simulink library "Ampere_Library"  (R2022b)
settings: Solver=FixedStepDiscrete  StartTime=0  StopTime=10.0  RelTol=1e-3  EnableMultiTasking=on
undefined symbols (not defined in the file or in its folder): A_INST_double, Dem_EventStatusType, ECU_AMBIENT_TEMPERATURE, SET_ECU_AMBIENT_TEMPERATURE, SlDemoSign, Std_ReturnType
libraries: simulink x13
(part 8 of 10)

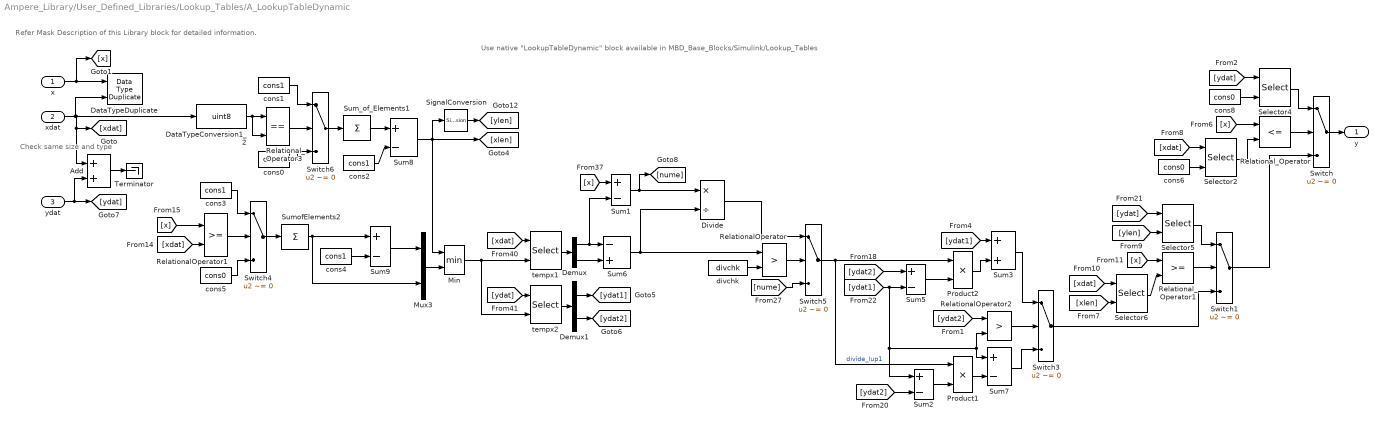
== system Ampere_Library/User_Defined_Libraries/Lookup_Tables/A_LookupTableDynamic ==
  note: Check same size and type
  note: Refer Mask Description of this Library block for detailed information.
  note: Use native "LookupTableDynamic" block available in MBD_Base_Blocks/Simulink/Lookup_Tables
  x : Inport
  xdat : Inport  Port=2
  ydat : Inport  Port=3
  Add : Sum  InputSameDT=on  RndMeth=Zero
  DataTypeConversion1_2 : DataTypeConversion  OutDataTypeStr=uint8
      settings: AttributesFormatString=SAT = %<SaturateOnIntegerOverflow>
  DataTypeDuplicate : DataTypeDuplicate
  Demux : Demux  Outputs=2
  Demux1 : Demux  Outputs=2
  Divide : Product  Inputs=*/  OutDataTypeStr=Inherit: Inherit via back propagation  RndMeth=Zero
      settings: AttributesFormatString=SAT = %<SaturateOnIntegerOverflow>\nDT = %<OutDataTypeStr>\n
  Min : MinMax  Inputs=2  InputSameDT=on  RndMeth=Zero  SaturateOnIntegerOverflow=on
      settings: AttributesFormatString=SAT = %<SaturateOnIntegerOverflow>
  Mux3 : Mux  Inputs=2
  Product1 : Product  OutDataTypeStr=Inherit: Inherit via back propagation  RndMeth=Zero
      settings: AttributesFormatString=SAT = %<SaturateOnIntegerOverflow>\nDT = %<OutDataTypeStr>\n
  Product2 : Product  OutDataTypeStr=Inherit: Inherit via back propagation  RndMeth=Zero
      settings: AttributesFormatString=SAT = %<SaturateOnIntegerOverflow>\nDT = %<OutDataTypeStr>\n
  RelationalOperator : RelationalOperator  Operator=>  OutDataTypeStr=boolean  RndMeth=Zero
  RelationalOperator1 : RelationalOperator  OutDataTypeStr=boolean  RndMeth=Zero
  RelationalOperator2 : RelationalOperator  Operator=>  OutDataTypeStr=boolean  RndMeth=Zero
  Relational_Operator : RelationalOperator  Operator=<=  OutDataTypeStr=boolean  RndMeth=Zero
  Relational_Operator1 : RelationalOperator  OutDataTypeStr=boolean  RndMeth=Zero
  Relational_Operator3 : RelationalOperator  Operator===  OutDataTypeStr=boolean  RndMeth=Zero
  Selector{2,4..6} (4 alike) : Selector  IndexMode=Zero-based  IndexOptions=Index vector (port)  Indices=SelIdx  OutputSizes=1
  SignalConversion : SignalConversion  OverrideOpt=off
  Sum{1..2,5,7} (4 alike) : Sum  Inputs=+-  InputSameDT=on  RndMeth=Zero
      settings: AttributesFormatString=SAT = %<SaturateOnIntegerOverflow>
  Sum3 : Sum  InputSameDT=on  RndMeth=Zero
      settings: AttributesFormatString=SAT = %<SaturateOnIntegerOverflow>
  Sum6 : Sum  Inputs=-+  InputSameDT=on  RndMeth=Zero
      settings: AttributesFormatString=SAT = %<SaturateOnIntegerOverflow>
  Sum8 : Sum  Inputs=+-  InputSameDT=on  RndMeth=Zero  SaturateOnIntegerOverflow=on
      settings: AttributesFormatString=SAT = %<SaturateOnIntegerOverflow>
  Sum9 : Sum  Inputs=+-  InputSameDT=on  RndMeth=Zero  SaturateOnIntegerOverflow=on
      settings: AttributesFormatString=SAT = %<SaturateOnIntegerOverflow>
  Sum_of_Elements1 : Sum  Inputs=+  InputSameDT=on  RndMeth=Zero  SaturateOnIntegerOverflow=on
      settings: AttributesFormatString=SAT = %<SaturateOnIntegerOverflow>
  SumofElements2 : Sum  Inputs=+  InputSameDT=on  RndMeth=Zero  SaturateOnIntegerOverflow=on
      settings: AttributesFormatString=SAT = %<SaturateOnIntegerOverflow>\n
  Switch{,1,3..6} (6 alike) : Switch  Criteria=u2 ~= 0  RndMeth=Zero  SaturateOnIntegerOverflow=off
      settings: AttributesFormatString=SAT = %<SaturateOnIntegerOverflow>
  Terminator : Terminator
  cons{0,5..6,8} (4 alike) : Constant  Value=cons0  OutDataTypeStr=uint8
      cons0 settings: AttributesFormatString=DT = %<OutDataTypeStr>
      cons5 settings: AttributesFormatString=DT = %<OutDataTypeStr>\n
      cons6 settings: AttributesFormatString=DT = %<OutDataTypeStr>\n
      cons8 settings: AttributesFormatString=DT = %<OutDataTypeStr>\n
  cons{1..4} (4 alike) : Constant  Value=cons1  OutDataTypeStr=uint8
      cons1 settings: AttributesFormatString=DT = %<OutDataTypeStr>
      cons2 settings: AttributesFormatString=DT = %<OutDataTypeStr>
      cons3 settings: AttributesFormatString=DT = %<OutDataTypeStr>\n
      cons4 settings: AttributesFormatString=DT = %<OutDataTypeStr>\n
  divchk : Constant  Value=divchk  OutDataTypeStr=Inherit: Inherit via back propagation
  tempx1 : Selector  IndexMode=Zero-based  IndexOptions=Index vector (port)  Indices=SelIdx  OutputSizes=2
  tempx2 : Selector  IndexMode=Zero-based  IndexOptions=Index vector (port)  Indices=SelIdx  OutputSizes=2
  y : Outport
  wires:
  Sum9/1 -> Mux3/1
  cons2/1 -> Sum8/2
  Sum_of_Elements1/1 -> Sum8/1
  SumofElements2/1 -> Sum9/1, Mux3/2
  Sum8/1 -> [xlen], SignalConversion/1, Min/1
  Relational_Operator/1 -> Switch/2
  Switch3/1 -> Switch1/3
  Sum2/1 -> Product1/2
  Sum7/1 -> Switch3/3
  Product1/1 -> Sum7/2
  Sum3/1 -> Switch3/1
  Switch5/1 -> Product2/1, Product1/1  "divide_lup1"
  Sum5/1 -> Product2/2
  [ydat2] -> Sum5/1
  RelationalOperator2/1 -> Switch3/2
  Divide/1 -> Switch5/1
  [ylen] -> Selector5/2
  [ydat] -> Selector5/1
  DataTypeConversion1_2/1 -> Relational_Operator3/2, Relational_Operator3/1
  Switch6/1 -> Sum_of_Elements1/1
  xdat/1 -> DataTypeConversion1_2/1, Add/1, [xdat], DataTypeDuplicate/2
  [xlen] -> Selector6/2
  [xdat] -> Selector6/1
  [ydat1] -> Sum5/2, Sum2/1, Sum7/1, RelationalOperator2/2
  [ydat2] -> Sum2/2
  Selector2/1 -> Relational_Operator/2
  cons6/1 -> Selector2/2
  [xdat] -> Selector2/1
  Sum6/1 -> RelationalOperator/1, Divide/2
  [nume] -> Switch5/3
  Sum1/1 -> [nume], Divide/1
  RelationalOperator/1 -> Switch5/2
  divchk/1 -> RelationalOperator/2
  Demux1/2 -> [ydat2]
  Demux1/1 -> [ydat1]
  Product2/1 -> Sum3/2
  [ydat1] -> Sum3/1
  cons8/1 -> Selector4/2
  tempx1/1 -> Demux/1
  Switch/1 -> y/1
  tempx2/1 -> Demux1/1
  Demux/2 -> Sum6/2
  Demux/1 -> Sum6/1, Sum1/2
  Selector5/1 -> Switch1/1
  [ydat] -> Selector4/1
  Selector4/1 -> Switch/1
  Selector6/1 -> Relational_Operator1/2
  [x] -> Relational_Operator/1
  [x] -> Relational_Operator1/1
  Relational_Operator1/1 -> Switch1/2
  Switch1/1 -> Switch/3
  Switch4/1 -> SumofElements2/1
  cons4/1 -> Sum9/2
  [x] -> RelationalOperator1/1
  [xdat] -> RelationalOperator1/2
  Min/1 -> tempx1/2, tempx2/2
  Mux3/1 -> Min/2
  RelationalOperator1/1 -> Switch4/2
  cons3/1 -> Switch4/1
  cons5/1 -> Switch4/3
  Relational_Operator3/1 -> Switch6/2
  cons1/1 -> Switch6/1
  cons0/1 -> Switch6/3
  x/1 -> [x], DataTypeDuplicate/1
  [x] -> Sum1/1
  [xdat] -> tempx1/1
  ydat/1 -> Add/2, [ydat]
  [ydat] -> tempx2/1
  SignalConversion/1 -> [ylen]
  [ydat2] -> RelationalOperator2/1
  Add/1 -> Terminator/1

== system Ampere_Library/User_Defined_Libraries/Lookup_Tables/A_SaturatedLookUpTable ==
  note: Resolution_system
  note: Refer Mask Description of this Library block for detailed information.
  note: Rounding_system
  in : Inport
  Abs1 : Abs  RndMeth=Zero  SaturateOnIntegerOverflow=off
  Constant : Constant  Value=Resolution  OutDataTypeStr=Inherit: Inherit via back propagation
  Constant1 : Constant  Value=RF5  OutDataTypeStr=Inherit: Inherit via back propagation
  Constant2 : Constant  Value=RF0  OutDataTypeStr=Inherit: Inherit via back propagation
  Constant3 : Constant  Value=RF1  OutDataTypeStr=Inherit: Inherit via back propagation
  Constant4 : Constant  Value=RF1  OutDataTypeStr=Inherit: Inherit via back propagation
  Constant5 : Constant  Value=RF0  OutDataTypeStr=Inherit: Inherit via back propagation
  Constant6 : Constant  Value=Resolution  OutDataTypeStr=Inherit: Inherit via back propagation
  DataTypeConversion3 : DataTypeConversion  SaturateOnIntegerOverflow=off
  DataTypeDuplicate : DataTypeDuplicate
  DataTypeDuplicate1 : DataTypeDuplicate
  OneD_Lookup_Table : Lookup_n-D  NumberOfTableDimensions=1  BreakpointsForDimension1=input_vector  Table=output_vector  ExtrapMethod=Clip  UseLastTableValue=on  OutDataTypeStr=Inherit: Inherit from 'Table data'  RndMeth=Zero
      settings: AttributesFormatString=Table = %<Table>\n X = %<BreakpointsForDimension1>\n
  Product : Product  Inputs=*/  InputSameDT=on  OutDataTypeStr=Inherit: Inherit via back propagation  RndMeth=Zero
  Product1 : Product  Inputs=**  InputSameDT=on  OutDataTypeStr=single  RndMeth=Zero
      settings: AttributesFormatString=DT = %<OutDataTypeStr>\n
  Product2 : Product  InputSameDT=on  OutDataTypeStr=uint32  RndMeth=Zero  SaturateOnIntegerOverflow=on
      settings: AttributesFormatString=SAT = %<SaturateOnIntegerOverflow>\n DT = %<OutDataTypeStr>\n
  RelationalOperator1 : RelationalOperator  OutDataTypeStr=boolean  RndMeth=Zero
  RelationalOperator4 : RelationalOperator  Operator=>  OutDataTypeStr=boolean  RndMeth=Zero
  Subtract10 : Sum  Inputs=-+  InputSameDT=on  OutDataTypeStr=Inherit: Inherit via back propagation  RndMeth=Zero
  Subtract4 : Sum  Inputs=--  InputSameDT=on  RndMeth=Zero
  Subtract9 : Sum  InputSameDT=on  RndMeth=Zero
  Switch1 : Switch  Criteria=u2 ~= 0  RndMeth=Zero  SaturateOnIntegerOverflow=off
  Switch10 : Switch  Criteria=u2 ~= 0  RndMeth=Zero  SaturateOnIntegerOverflow=off
  out : Outport
  wires:
  in/1 -> OneD_Lookup_Table/1
  Product1/1 -> out/1
  Switch1/1 -> Subtract4/2, Subtract9/2  "GreaterDcon"
  RelationalOperator1/1 -> Switch1/2
  Constant1/1 -> RelationalOperator1/2
  [int_out] -> Subtract9/1
  [Check] -> Switch10/2
  Subtract4/1 -> Switch10/3
  [int_out] -> Subtract4/1
  RelationalOperator4/1 -> [Check]
  DataTypeConversion3/1 -> Subtract10/1, [int_out]
  Product2/1 -> DataTypeConversion3/1
  Constant2/1 -> RelationalOperator4/2
  Product/1 -> RelationalOperator4/1, Abs1/1, DataTypeDuplicate/2
  Constant3/1 -> Product2/1
  Abs1/1 -> Subtract10/2, Product2/2
  Subtract10/1 -> DataTypeDuplicate1/1, RelationalOperator1/1  "Difference"
  Subtract9/1 -> Switch10/1
  Constant5/1 -> Switch1/3
  Switch10/1 -> Product1/1
  OneD_Lookup_Table/1 -> DataTypeDuplicate/1, Product/1
  Constant/1 -> Product/2
  Constant6/1 -> Product1/2
  Constant4/1 -> DataTypeDuplicate1/2, Switch1/1

== system Ampere_Library/User_Defined_Libraries/Lookup_Tables/A_Sine ==
  note: Refer Mask Description of this Library block for detailed information.
  u : Inport
  Amp1 : Sum  Inputs=-+  InputSameDT=on  RndMeth=Zero  SaturateOnIntegerOverflow=on  LockScale=on
      settings: AttributesFormatString=SAT = %<SaturateOnIntegerOverflow>
  Amp50 : Sum  Inputs=+-  InputSameDT=on  RndMeth=Zero  SaturateOnIntegerOverflow=on  LockScale=on
      settings: AttributesFormatString=SAT = %<SaturateOnIntegerOverflow>
  CONS_M1 : Constant  Value=Cons_M1  OutDataTypeStr=int8
      settings: AttributesFormatString=DT = %<OutDataTypeStr>\n
  CONS_P25 : Constant  Value=Cons_P25  OutDataTypeStr=Inherit: Inherit via back propagation
  CONS_P5 : Constant  Value=Cons_P5  OutDataTypeStr=Inherit: Inherit via back propagation
  DataTypeConversion : DataTypeConversion  OutDataTypeStr=fixdt(0, OutputWordLength, OutputWordLength)
      settings: AttributesFormatString=|
      | SAT = %<SaturateOnIntegerOverflow>
      | DT = %<OutDataTypeStr>
  LookupTable1_D : Lookup_n-D  NumberOfTableDimensions=1  BreakpointsForDimension1=k  BeginIndexSearchUsingPreviousIndexResult=on  Table=b  ExtrapMethod=Clip  UseLastTableValue=on  OutDataTypeStr=fixdt(1, OutputWordLength, OutputFracLength)  RndMeth=Zero  SaturateOnIntegerOverflow=on  FractionDataTypeStr=double
      settings: AttributesFormatString=Table = %<Table>\n X = %<BreakpointsForDimension1>\n
  Product : Product  OutDataTypeStr=Inherit: Inherit via back propagation  RndMeth=Zero  SaturateOnIntegerOverflow=on
      settings: AttributesFormatString=SAT = %<SaturateOnIntegerOverflow>\n
  Relational_Operator1 : RelationalOperator  Operator=<=  OutDataTypeStr=boolean  RndMeth=Zero
  Relational_Operator3 : RelationalOperator  Operator=<=  OutDataTypeStr=boolean  RndMeth=Zero
  Switch1 : Switch  Criteria=u2 ~= 0  RndMeth=Zero
      settings: AttributesFormatString=SAT = %<SaturateOnIntegerOverflow>
  Switch2 : Switch  Criteria=u2 ~= 0  RndMeth=Zero
      settings: AttributesFormatString=SAT = %<SaturateOnIntegerOverflow>
  Switch4 : Switch  Criteria=u2 ~= 0  RndMeth=Zero
      settings: AttributesFormatString=SAT = %<SaturateOnIntegerOverflow>
  y : Outport
  wires:
  CONS_M1/1 -> Product/2
  Product/1 -> Switch2/3
  [IniIO] -> Amp50/1
  DataTypeConversion/1 -> Switch1/1, Relational_Operator1/1, [IniIO]
  LookupTable1_D/1 -> Product/1, Switch2/1
  Switch4/1 -> LookupTable1_D/1
  CONS_P5/1 -> Amp1/2, Relational_Operator1/2, Amp50/2
  Switch2/1 -> y/1
  [lespoint5] -> Switch2/2
  Amp1/1 -> Switch4/3
  Relational_Operator3/1 -> Switch4/2
  CONS_P25/1 -> Relational_Operator3/2
  Switch1/1 -> Amp1/1, Relational_Operator3/1, Switch4/1
  Amp50/1 -> Switch1/3
  u/1 -> DataTypeConversion/1
  Relational_Operator1/1 -> [lespoint5], Switch1/2

== system Ampere_Library/User_Defined_Libraries/Math_Operations/A_ADivB ==
  note: Refer Mask Description of this Library block for detailed information.
  A : Inport
  B : Inport  Port=2
  Abs1 : Abs  RndMeth=Zero  SaturateOnIntegerOverflow=off
      settings: AttributesFormatString=SAT = %<SaturateOnIntegerOverflow>
  Divide : Product  Inputs=*/  OutDataTypeStr=Inherit: Inherit via back propagation  RndMeth=Zero
      settings: AttributesFormatString=SAT = %<SaturateOnIntegerOverflow>\n
  RelationalOperator : RelationalOperator  Operator=>  OutDataTypeStr=boolean  RndMeth=Zero
  Switch : Switch  Criteria=u2 ~= 0  RndMeth=Zero  SaturateOnIntegerOverflow=off
      settings: AttributesFormatString=SAT = %<SaturateOnIntegerOverflow>
  divbyzval : Constant  Value=divbyzval  OutDataTypeStr=Inherit: Inherit via back propagation
  tol : Constant  Value=tol  OutDataTypeStr=Inherit: Inherit via back propagation
  AdivB : Outport
  wires:
  divbyzval/1 -> Switch/3
  tol/1 -> RelationalOperator/2
  A/1 -> Divide/1
  Abs1/1 -> RelationalOperator/1
  B/1 -> Abs1/1, Switch/1
  Divide/1 -> AdivB/1
  RelationalOperator/1 -> Switch/2
  Switch/1 -> Divide/2

== system Ampere_Library/User_Defined_Libraries/Math_Operations/A_DivisionByZero ==
  note: Refer Mask Description of this Library block for detailed information.
  den : Inport
  num : Inport  Port=2
  default : Inport  Port=3
  Abs1 : Abs  RndMeth=Zero  SaturateOnIntegerOverflow=off
      settings: AttributesFormatString=SAT = %<SaturateOnIntegerOverflow>
  Den_Tol : Constant  Value=Den_Tol  OutDataTypeStr=Inherit: Inherit via back propagation
  Divide : Product  Inputs=*/  OutDataTypeStr=Inherit: Inherit via back propagation  RndMeth=Zero
      settings: AttributesFormatString=SAT = %<SaturateOnIntegerOverflow>\n
  RelationalOperator : RelationalOperator  Operator=>  OutDataTypeStr=boolean  RndMeth=Zero
  Switch : Switch  Criteria=u2 ~= 0  RndMeth=Zero  SaturateOnIntegerOverflow=off
      settings: AttributesFormatString=SAT = %<SaturateOnIntegerOverflow>
  res : Outport
  wires:
  default/1 -> Switch/3
  Abs1/1 -> RelationalOperator/1
  den/1 -> Divide/2, Abs1/1
  Switch/1 -> res/1
  Den_Tol/1 -> RelationalOperator/2
  Divide/1 -> Switch/1
  RelationalOperator/1 -> Switch/2
  num/1 -> Divide/1

== system Ampere_Library/User_Defined_Libraries/Math_Operations/A_Modulo ==
  note: Unused data depending
      | of mask configuration
  note: Refer Mask Description of this Library block for detailed information.
  note: GotoTag updated through mask callback
  X : Inport
  Y : Inport  Port=2
  Abs1 : Abs  RndMeth=Zero  SaturateOnIntegerOverflow=off
      settings: AttributesFormatString=SAT = %<SaturateOnIntegerOverflow>
  Abs2 : Abs  RndMeth=Zero  SaturateOnIntegerOverflow=off
      settings: AttributesFormatString=SAT = %<SaturateOnIntegerOverflow>
  Add1 : Sum  Inputs=+-  InputSameDT=on  RndMeth=Zero
      settings: AttributesFormatString=SAT = %<SaturateOnIntegerOverflow>
  Add2 : Sum  Inputs=+-  InputSameDT=on  RndMeth=Zero
      settings: AttributesFormatString=SAT = %<SaturateOnIntegerOverflow>\n
  DataTypeDuplicate : DataTypeDuplicate
  Divide : Product  Inputs=*/  OutDataTypeStr=InternalDataType  RndMeth=Zero  SaturateOnIntegerOverflow=on
      settings: AttributesFormatString=SAT = %<SaturateOnIntegerOverflow>\n DT = %<OutDataTypeStr>\n
  LogicalOperator1 : Logic  OutDataTypeStr=boolean
  Product1 : Product  OutDataTypeStr=Inherit: Inherit via back propagation  RndMeth=Zero
      settings: AttributesFormatString=SAT = %<SaturateOnIntegerOverflow>
  Product2 : Product  OutDataTypeStr=Inherit: Inherit via back propagation  RndMeth=Zero
      settings: AttributesFormatString=SAT = %<SaturateOnIntegerOverflow>
  RelationalOperator1 : RelationalOperator  Operator=>  OutDataTypeStr=boolean  RndMeth=Zero
  RelationalOperator2 : RelationalOperator  Operator=>  OutDataTypeStr=boolean  RndMeth=Zero
  RelationalOperator5 : RelationalOperator  Operator=<  OutDataTypeStr=boolean  RndMeth=Zero
  RelationalOperator6 : RelationalOperator  Operator=<  OutDataTypeStr=boolean  RndMeth=Zero
  Sign : Signum
  Switch : Switch  Criteria=u2 ~= 0  RndMeth=Zero  SaturateOnIntegerOverflow=off
      settings: AttributesFormatString=SAT = %<SaturateOnIntegerOverflow>
  Switch4 : Switch  Criteria=u2 ~= 0  RndMeth=Zero  SaturateOnIntegerOverflow=off
      settings: AttributesFormatString=SAT = %<SaturateOnIntegerOverflow>
  Terminator1 : Terminator
  Terminator2 : Terminator
  XOR : Logic  Operator=XOR  OutDataTypeStr=boolean
  cmpTol : Constant  Value=cmpTol  OutDataTypeStr=Inherit: Inherit via back propagation
  cmpZero : Constant  Value=cmpZero  OutDataTypeStr=Inherit: Inherit via back propagation
  constOne : Constant  Value=constOne  OutDataTypeStr=uint8
      settings: AttributesFormatString=DT = %<OutDataTypeStr>\n
  M : Outport
  wires:
  Add2/1 -> Switch4/1
  RelationalOperator1/1 -> Switch/2
  cmpZero/1 -> RelationalOperator5/2, RelationalOperator2/2, RelationalOperator6/2
  Add1/1 -> Add2/2, Switch4/3, RelationalOperator2/1
  [absY] -> Add2/1
  Abs1/1 -> Add1/1, Divide/1
  [X] -> Switch/3
  [Y] -> RelationalOperator5/1
  Product2/1 -> Add1/2
  LogicalOperator1/1 -> Switch4/2
  Sign/1 -> [Mulconst]
  [absY] -> RelationalOperator1/1
  cmpTol/1 -> RelationalOperator1/2
  Divide/1 -> Product2/1
  RelationalOperator2/1 -> LogicalOperator1/2
  XOR/1 -> LogicalOperator1/1
  RelationalOperator5/1 -> XOR/2
  Product1/1 -> Switch/1
  [constone] -> Product1/2
  [X] -> RelationalOperator6/1
  Switch/1 -> M/1
  constOne/1 -> [constone]
  [constone] -> Terminator1/1
  Y/1 -> [Y], Abs2/1, Sign/1, DataTypeDuplicate/2
  [Mulconst] -> Terminator2/1
  X/1 -> [X], Abs1/1, DataTypeDuplicate/1
  RelationalOperator6/1 -> XOR/1
  Abs2/1 -> [absY], Divide/2, Product2/2
  Switch4/1 -> Product1/1

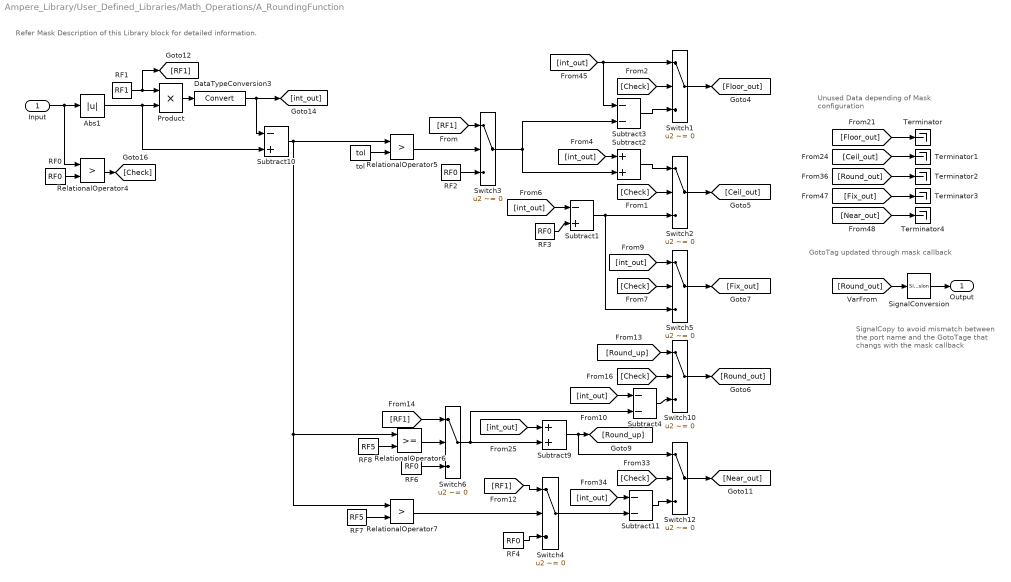
== system Ampere_Library/User_Defined_Libraries/Math_Operations/A_RoundingFunction ==
  note: GotoTag updated through mask callback
  note: Unused Data depending of
      | Mask configuration
  note: SignalCopy to avoid mismatch between the port name and the GotoTage that changs with the mask callback
  note: Refer Mask Description of this Library block for detailed information.
  Input : Inport
  Abs1 : Abs  RndMeth=Zero  SaturateOnIntegerOverflow=off
  DataTypeConversion3 : DataTypeConversion  SaturateOnIntegerOverflow=off
  Product : Product  OutDataTypeStr=uint32  RndMeth=Zero  SaturateOnIntegerOverflow=on
      settings: AttributesFormatString=SAT = %<SaturateOnIntegerOverflow>\n DT = %<OutDataTypeStr>\n
  RF{0,2..4,6} (5 alike) : Constant  Value=RF0  OutDataTypeStr=Inherit: Inherit via back propagation
  RF1 : Constant  Value=RF1  OutDataTypeStr=Inherit: Inherit via back propagation
  RF7 : Constant  Value=RF5  OutDataTypeStr=Inherit: Inherit via back propagation
  RF8 : Constant  Value=RF5  OutDataTypeStr=Inherit: Inherit via back propagation
  RelationalOperator4 : RelationalOperator  Operator=>  OutDataTypeStr=boolean  RndMeth=Zero
  RelationalOperator5 : RelationalOperator  Operator=>  OutDataTypeStr=boolean  RndMeth=Zero
  RelationalOperator6 : RelationalOperator  OutDataTypeStr=boolean  RndMeth=Zero
  RelationalOperator7 : RelationalOperator  Operator=>  OutDataTypeStr=boolean  RndMeth=Zero
  SignalConversion : SignalConversion  OverrideOpt=off
  Subtract1 : Sum  Inputs=-+  InputSameDT=on  RndMeth=Zero
  Subtract10 : Sum  Inputs=-+  InputSameDT=on  RndMeth=Zero
  Subtract11 : Sum  Inputs=--  InputSameDT=on  RndMeth=Zero
  Subtract2 : Sum  InputSameDT=on  RndMeth=Zero
  Subtract3 : Sum  Inputs=--  InputSameDT=on  RndMeth=Zero
  Subtract4 : Sum  Inputs=--  InputSameDT=on  RndMeth=Zero
  Subtract9 : Sum  InputSameDT=on  RndMeth=Zero
  Switch{1..6,10,12} (8 alike) : Switch  Criteria=u2 ~= 0  RndMeth=Zero  SaturateOnIntegerOverflow=off
  Terminator{,1..4} (5 alike) : Terminator
  tol : Constant  Value=tol  OutDataTypeStr=Inherit: Inherit via back propagation
  Output : Outport
  wires:
  [RF1] -> Switch6/1
  RelationalOperator6/1 -> Switch6/2
  RF6/1 -> Switch6/3
  [RF1] -> Switch4/1
  RelationalOperator7/1 -> Switch4/2
  RF4/1 -> Switch4/3
  [RF1] -> Switch3/1
  RelationalOperator5/1 -> Switch3/2
  RF2/1 -> Switch3/3
  Switch3/1 -> Subtract3/2, Subtract2/2
  [Check] -> Switch12/2
  Subtract11/1 -> Switch12/3
  [int_out] -> Subtract11/1
  Switch4/1 -> Subtract11/2
  RF7/1 -> RelationalOperator7/2
  [int_out] -> Subtract9/1
  Switch6/1 -> Subtract9/2, Subtract4/2
  Subtract10/1 -> RelationalOperator7/1, RelationalOperator6/1, RelationalOperator5/1
  RF8/1 -> RelationalOperator6/2
  [Round_out] -> SignalConversion/1
  [Near_out] -> Terminator4/1
  [Fix_out] -> Terminator3/1
  [Round_out] -> Terminator2/1
  [Ceil_out] -> Terminator1/1
  [Floor_out] -> Terminator/1
  [int_out] -> Subtract3/1, Switch1/1
  RF3/1 -> Subtract1/2
  Switch10/1 -> [Round_out]
  Switch5/1 -> [Fix_out]
  [Check] -> Switch10/2
  Subtract4/1 -> Switch10/3
  [Round_up] -> Switch10/1
  [Check] -> Switch5/2
  [int_out] -> Switch5/1
  [int_out] -> Subtract1/1
  Subtract1/1 -> Switch5/3, Switch2/3
  Switch1/1 -> [Floor_out]
  Switch2/1 -> [Ceil_out]
  [int_out] -> Subtract2/1
  Subtract2/1 -> Switch2/1
  [Check] -> Switch2/2
  [Check] -> Switch1/2
  Switch12/1 -> [Near_out]
  Subtract3/1 -> Switch1/3
  RelationalOperator4/1 -> [Check]
  DataTypeConversion3/1 -> [int_out], Subtract10/1
  Product/1 -> DataTypeConversion3/1
  RF0/1 -> RelationalOperator4/2
  Input/1 -> Abs1/1, RelationalOperator4/1
  RF1/1 -> Product/1, [RF1]
  Abs1/1 -> Subtract10/2, Product/2
  tol/1 -> RelationalOperator5/2
  Subtract9/1 -> Switch12/1, [Round_up]
  [int_out] -> Subtract4/1
  SignalConversion/1 -> Output/1

== system Ampere_Library/User_Defined_Libraries/Math_Operations/A_SquareRoot ==
  note: Refer Mask Description of this Library block for detailed information.
  In : Inport
  RelationalOperator : RelationalOperator  Operator=<  OutDataTypeStr=boolean  RndMeth=Zero
  Switch : Switch  Criteria=u2 ~= 0  RndMeth=Zero  SaturateOnIntegerOverflow=off
      settings: AttributesFormatString=SAT = %<SaturateOnIntegerOverflow>
  While_Iterator : Subsystem  TreatAsAtomicUnit=on
      settings: RTWSystemCode=Inline
  cmpTol : Constant  Value=cmpTol  OutDataTypeStr=Inherit: Inherit via back propagation
  constZero : Constant  DisableCoverage=on  Value=constZero  OutDataTypeStr=Inherit: Inherit via back propagation  PreserveConstantTs=on
  Out : Outport
  wires:
  Switch/1 -> Out/1
  constZero/1 -> Switch/1
  RelationalOperator/1 -> Switch/2
  While_Iterator/1(Out) -> Switch/3
  cmpTol/1 -> RelationalOperator/2
  In/1 -> RelationalOperator/1, While_Iterator/1(In)

== system Ampere_Library/User_Defined_Libraries/Math_Operations/A_XSquare ==
  note: Unused data depending
      | of the mask configuration
  note: Min/Max updated via mask
  note: From Tag updated via mask
  note: Refer Mask Description of this Library block for detailed information.
  note: DT updated via mask
  In : Inport
  Product : Product  InputSameDT=on  OutDataTypeStr=double  RndMeth=Zero
      settings: AttributesFormatString=DT = %<OutDataTypeStr>\n
  Saturation1 : Saturate  UpperLimit=XS_double_Max  LowerLimit=XS_double_Min  RndMeth=Zero
      settings: AttributesFormatString="Max =  %<UpperLimit>\\n Min = %<LowerLimit> \\n"
  Terminator : Terminator
  Terminator1 : Terminator
  Out : Outport
  wires:
  Product/1 -> Out/1
  [sq_input] -> Product/1, Product/2
  In/1 -> Saturation1/1, [In]
  Saturation1/1 -> [sq_input]
  [sq_input] -> Terminator/1
  [In] -> Terminator1/1

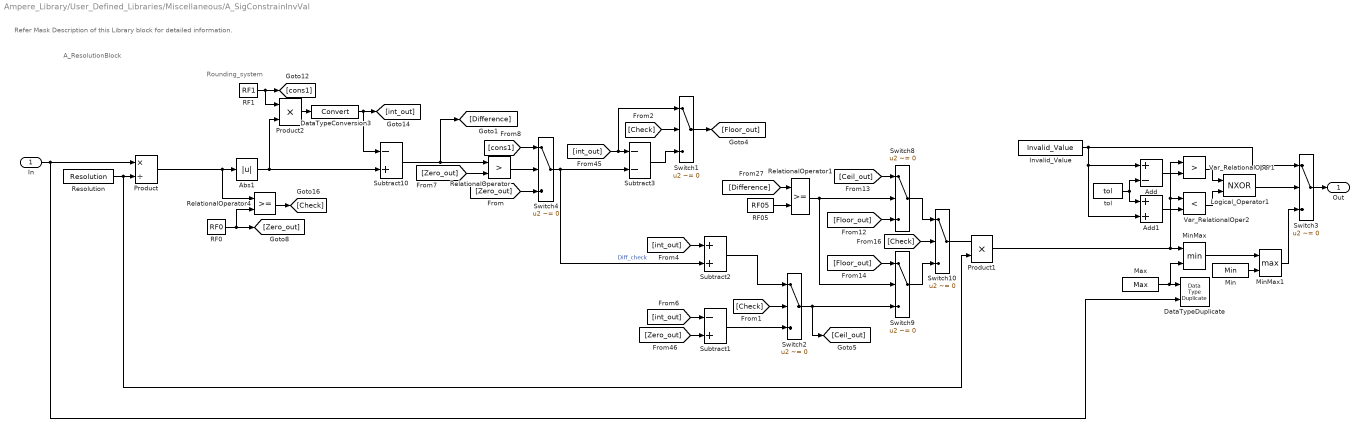
== system Ampere_Library/User_Defined_Libraries/Miscellaneous/A_SigConstrainInvVal ==
  note: Rounding_system
  note: Refer Mask Description of this Library block for detailed information.
  note: A_ResolutionBlock
  In : Inport
  Abs1 : Abs  RndMeth=Zero  SaturateOnIntegerOverflow=off
      settings: AttributesFormatString=SAT = %<SaturateOnIntegerOverflow>
  Add : Sum  Inputs=+-  InputSameDT=on  RndMeth=Zero
  Add1 : Sum  InputSameDT=on  RndMeth=Zero
  DataTypeConversion3 : DataTypeConversion  SaturateOnIntegerOverflow=off
      settings: AttributesFormatString=SAT = %<SaturateOnIntegerOverflow>
  DataTypeDuplicate : DataTypeDuplicate
  Invalid_Value : Constant  Value=Invalid_Value  OutDataTypeStr=Inherit: Inherit via back propagation
  Logical_Operator1 : Logic  Operator=NXOR  OutDataTypeStr=boolean
  Max : Constant  Value=Max  OutDataTypeStr=Inherit: Inherit via back propagation
  Min : Constant  Value=Min  OutDataTypeStr=Inherit: Inherit via back propagation
  MinMax : MinMax  Inputs=2  InputSameDT=on  RndMeth=Zero
  MinMax1 : MinMax  Function=max  Inputs=2  InputSameDT=on  RndMeth=Zero
  Product : Product  Inputs=*/  InputSameDT=on  OutDataTypeStr=Inherit: Inherit via back propagation  RndMeth=Zero
      settings: AttributesFormatString=SAT = %<SaturateOnIntegerOverflow>\n Out DT = %<OutDataTypeStr>\n
  Product1 : Product  Inputs=**  InputSameDT=on  OutDataTypeStr=double  RndMeth=Zero
      settings: AttributesFormatString=SAT = %<SaturateOnIntegerOverflow>\n DT = %<OutDataTypeStr>\n
  Product2 : Product  OutDataTypeStr=uint32  RndMeth=Zero  SaturateOnIntegerOverflow=on
      settings: AttributesFormatString=SAT = %<SaturateOnIntegerOverflow>\n DT = %<OutDataTypeStr>\n
  RF0 : Constant  Value=RF0
  RF05 : Constant  Value=RF05
  RF1 : Constant  Value=RF1
  RelationalOperator : RelationalOperator  Operator=>  OutDataTypeStr=boolean  RndMeth=Zero
  RelationalOperator1 : RelationalOperator  OutDataTypeStr=boolean  RndMeth=Zero
  RelationalOperator4 : RelationalOperator  OutDataTypeStr=boolean  RndMeth=Zero
  Resolution : Constant  Value=Resolution  OutDataTypeStr=Inherit: Inherit via back propagation
  Subtract1 : Sum  Inputs=-+  InputSameDT=on  RndMeth=Zero
      settings: AttributesFormatString=SAT = %<SaturateOnIntegerOverflow>\n Out DT = %<OutDataTypeStr>\n
  Subtract10 : Sum  Inputs=-+  InputSameDT=on  RndMeth=Zero
      settings: AttributesFormatString=SAT = %<SaturateOnIntegerOverflow>\n Out DT = %<OutDataTypeStr>\n
  Subtract2 : Sum  InputSameDT=on  RndMeth=Zero
      settings: AttributesFormatString=SAT = %<SaturateOnIntegerOverflow>\n Out DT = %<OutDataTypeStr>\n
  Subtract3 : Sum  Inputs=--  InputSameDT=on  RndMeth=Zero
      settings: AttributesFormatString=SAT = %<SaturateOnIntegerOverflow>\n Out DT = %<OutDataTypeStr>\n
  Switch{1..4,8..10} (7 alike) : Switch  Criteria=u2 ~= 0  RndMeth=Zero  SaturateOnIntegerOverflow=off
  Var_RelationalOper1 : RelationalOperator  Operator=>  OutDataTypeStr=boolean  RndMeth=Zero
  Var_RelationalOper2 : RelationalOperator  Operator=<  OutDataTypeStr=boolean  RndMeth=Zero
  tol : Constant  Value=tol  OutDataTypeStr=Inherit: Inherit via back propagation
  Out : Outport
  wires:
  Switch10/1 -> Product1/1
  In/1 -> Product/1, DataTypeDuplicate/2
  Resolution/1 -> Product/2, Product1/2
  [Zero_out] -> Switch4/3
  [cons1] -> Switch4/1
  [Zero_out] -> RelationalOperator/2
  Subtract10/1 -> [Difference], RelationalOperator/1
  RelationalOperator4/1 -> [Check]
  DataTypeConversion3/1 -> Subtract10/1, [int_out]
  Product2/1 -> DataTypeConversion3/1
  RF0/1 -> [Zero_out], RelationalOperator4/2
  Product/1 -> Abs1/1, RelationalOperator4/1
  RF1/1 -> Product2/1, [cons1]
  Abs1/1 -> Subtract10/2, Product2/2
  RelationalOperator1/1 -> Switch9/2, Switch8/2
  [Ceil_out] -> Switch8/1
  [Floor_out] -> Switch8/3
  [Floor_out] -> Switch9/1
  Switch2/1 -> [Ceil_out], Switch9/3
  Switch8/1 -> Switch10/1
  Switch9/1 -> Switch10/3
  [Check] -> Switch10/2
  [Difference] -> RelationalOperator1/1
  RF05/1 -> RelationalOperator1/2
  Subtract3/1 -> Switch1/3
  [Check] -> Switch1/2
  [Check] -> Switch2/2
  Subtract2/1 -> Switch2/1
  [int_out] -> Subtract2/1
  Switch1/1 -> [Floor_out]
  Subtract1/1 -> Switch2/3
  [int_out] -> Subtract1/1
  [Zero_out] -> Subtract1/2
  [int_out] -> Subtract3/1, Switch1/1
  RelationalOperator/1 -> Switch4/2
  Switch4/1 -> Subtract3/2, Subtract2/2  "Diff_check"
  Min/1 -> MinMax1/2
  MinMax/1 -> MinMax1/1
  Invalid_Value/1 -> Switch3/1, Add1/2, Add/1
  Add1/1 -> Var_RelationalOper2/2
  Var_RelationalOper2/1 -> Logical_Operator1/2
  tol/1 -> Add/2, Add1/1
  Add/1 -> Var_RelationalOper1/2
  Product1/1 -> MinMax/1, Var_RelationalOper1/1, Var_RelationalOper2/1
  Var_RelationalOper1/1 -> Logical_Operator1/1
  Max/1 -> MinMax/2, DataTypeDuplicate/1
  MinMax1/1 -> Switch3/3
  Logical_Operator1/1 -> Switch3/2
  Switch3/1 -> Out/1

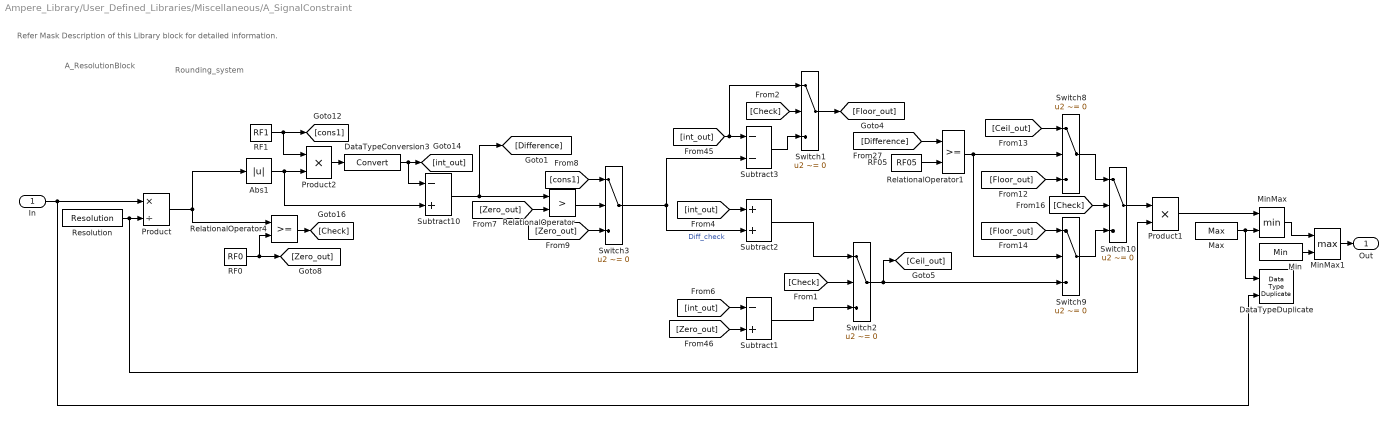
== system Ampere_Library/User_Defined_Libraries/Miscellaneous/A_SignalConstraint ==
  note: A_ResolutionBlock
  note: Refer Mask Description of this Library block for detailed information.
  note: Rounding_system
  In : Inport
  Abs1 : Abs  RndMeth=Zero  SaturateOnIntegerOverflow=off
      settings: AttributesFormatString=SAT = %<SaturateOnIntegerOverflow>
  DataTypeConversion3 : DataTypeConversion  SaturateOnIntegerOverflow=off
      settings: AttributesFormatString=SAT = %<SaturateOnIntegerOverflow>
  DataTypeDuplicate : DataTypeDuplicate
  Max : Constant  Value=Max  OutDataTypeStr=Inherit: Inherit via back propagation
  Min : Constant  Value=Min  OutDataTypeStr=Inherit: Inherit via back propagation
  MinMax : MinMax  Inputs=2  InputSameDT=on  RndMeth=Zero
  MinMax1 : MinMax  Function=max  Inputs=2  InputSameDT=on  RndMeth=Zero
  Product : Product  Inputs=*/  InputSameDT=on  OutDataTypeStr=Inherit: Inherit via back propagation  RndMeth=Zero
      settings: AttributesFormatString=SAT = %<SaturateOnIntegerOverflow>\nDT = %<OutDataTypeStr>\n
  Product1 : Product  Inputs=**  InputSameDT=on  OutDataTypeStr=double  RndMeth=Zero
      settings: AttributesFormatString=SAT = %<SaturateOnIntegerOverflow>\n DT = %<OutDataTypeStr>\n
  Product2 : Product  OutDataTypeStr=uint32  RndMeth=Zero  SaturateOnIntegerOverflow=on
      settings: AttributesFormatString=SAT = %<SaturateOnIntegerOverflow>\n DT = %<OutDataTypeStr>\n
  RF0 : Constant  Value=RF0  OutDataTypeStr=Inherit: Inherit via back propagation
  RF05 : Constant  Value=RF05  OutDataTypeStr=Inherit: Inherit via back propagation
  RF1 : Constant  Value=RF1  OutDataTypeStr=Inherit: Inherit via back propagation
  RelationalOperator : RelationalOperator  Operator=>  OutDataTypeStr=boolean  RndMeth=Zero
  RelationalOperator1 : RelationalOperator  OutDataTypeStr=boolean  RndMeth=Zero
  RelationalOperator4 : RelationalOperator  OutDataTypeStr=boolean  RndMeth=Zero
  Resolution : Constant  Value=Resolution  OutDataTypeStr=Inherit: Inherit via back propagation
  Subtract1 : Sum  Inputs=-+  InputSameDT=on  OutDataTypeStr=Inherit: Inherit via back propagation  RndMeth=Zero
      settings: AttributesFormatString=SAT = %<SaturateOnIntegerOverflow>\n Out DT = %<OutDataTypeStr>\n
  Subtract10 : Sum  Inputs=-+  InputSameDT=on  OutDataTypeStr=Inherit: Inherit via back propagation  RndMeth=Zero
      settings: AttributesFormatString=SAT = %<SaturateOnIntegerOverflow>\n Out DT = %<OutDataTypeStr>\n
  Subtract2 : Sum  InputSameDT=on  OutDataTypeStr=Inherit: Inherit via back propagation  RndMeth=Zero
      settings: AttributesFormatString=SAT = %<SaturateOnIntegerOverflow>\n Out DT = %<OutDataTypeStr>\n
  Subtract3 : Sum  Inputs=--  InputSameDT=on  OutDataTypeStr=Inherit: Inherit via back propagation  RndMeth=Zero
      settings: AttributesFormatString=SAT = %<SaturateOnIntegerOverflow>\n Out DT = %<OutDataTypeStr>\n
  Switch{1..3,8..10} (6 alike) : Switch  Criteria=u2 ~= 0  RndMeth=Zero  SaturateOnIntegerOverflow=off
  Out : Outport
  wires:
  Max/1 -> MinMax/2, DataTypeDuplicate/1
  MinMax1/1 -> Out/1
  Product1/1 -> MinMax/1
  Min/1 -> MinMax1/2
  MinMax/1 -> MinMax1/1
  [Zero_out] -> Switch3/3
  [cons1] -> Switch3/1
  [Zero_out] -> RelationalOperator/2
  Subtract10/1 -> RelationalOperator/1, [Difference]
  RelationalOperator4/1 -> [Check]
  DataTypeConversion3/1 -> Subtract10/1, [int_out]
  Product2/1 -> DataTypeConversion3/1
  RF0/1 -> RelationalOperator4/2, [Zero_out]
  Product/1 -> Abs1/1, RelationalOperator4/1
  RF1/1 -> Product2/1, [cons1]
  Abs1/1 -> Product2/2, Subtract10/2
  RelationalOperator1/1 -> Switch9/2, Switch8/2
  [Ceil_out] -> Switch8/1
  [Floor_out] -> Switch8/3
  [Floor_out] -> Switch9/1
  Switch2/1 -> Switch9/3, [Ceil_out]
  Switch8/1 -> Switch10/1
  Switch9/1 -> Switch10/3
  [Check] -> Switch10/2
  [Difference] -> RelationalOperator1/1
  RF05/1 -> RelationalOperator1/2
  Subtract3/1 -> Switch1/3
  [Check] -> Switch1/2
  [Check] -> Switch2/2
  Subtract2/1 -> Switch2/1
  [int_out] -> Subtract2/1
  Switch1/1 -> [Floor_out]
  Subtract1/1 -> Switch2/3
  [int_out] -> Subtract1/1
  [Zero_out] -> Subtract1/2
  [int_out] -> Switch1/1, Subtract3/1
  RelationalOperator/1 -> Switch3/2
  Switch3/1 -> Subtract2/2, Subtract3/2  "Diff_check"
  Switch10/1 -> Product1/1
  In/1 -> DataTypeDuplicate/2, Product/1
  Resolution/1 -> Product1/2, Product/2

== system Ampere_Library/User_Defined_Libraries/Signal_Routing/A_DataTypeDuplicate ==
  note: Refer Mask Description of this Library block for detailed information.
  note: Use native "DataTypeDuplicate" block available in MBD_Base_Blocks/Simulink/Signal_Attributes
  In1 : Inport
  In2 : Inport  Port=2
  In3 : Inport  Port=3
  Mux : Mux  Inputs=3
  Terminator : Terminator
  wires:
  In3/1 -> Mux/3
  In2/1 -> Mux/2
  In1/1 -> Mux/1
  Mux/1 -> Terminator/1

== system Ampere_Library/User_Defined_Libraries/Signal_Routing/A_DefaultValueSwitch ==
  note: Refer Mask Description of this Library block for detailed information.
  U : Inport
  Add : Sum  Inputs=+-  InputSameDT=on  RndMeth=Zero
      settings: AttributesFormatString=SAT = %<SaturateOnIntegerOverflow>
  Add1 : Sum  InputSameDT=on  RndMeth=Zero
      settings: AttributesFormatString=SAT = %<SaturateOnIntegerOverflow>
  DataTypeDuplicate : DataTypeDuplicate
  DefaultValue : Constant  Value=DefaultValue  OutDataTypeStr=Inherit: Inherit via back propagation
  InvalidValue : Constant  Value=InvalidValue  OutDataTypeStr=Inherit: Inherit via back propagation
  Logical_Operator1 : Logic  Operator=NOT  OutDataTypeStr=boolean
  Logical_Operator12 : Logic  Operator=XOR  OutDataTypeStr=boolean
  Switch2 : Switch  Criteria=u2 ~= 0  RndMeth=Zero  SaturateOnIntegerOverflow=off
      settings: AttributesFormatString=SAT = %<SaturateOnIntegerOverflow>
  Var_RelationalOper1 : RelationalOperator  Operator=>  OutDataTypeStr=boolean  RndMeth=Zero
  Var_RelationalOper2 : RelationalOperator  Operator=<  OutDataTypeStr=boolean  RndMeth=Zero
  tol : Constant  Value=tol  OutDataTypeStr=Inherit: Inherit via back propagation
  tol1 : Constant  Value=tol  OutDataTypeStr=Inherit: Inherit via back propagation
  Y : Outport
  wires:
  Add/1 -> Var_RelationalOper1/2
  DefaultValue/1 -> Switch2/1
  Var_RelationalOper2/1 -> Logical_Operator12/2
  tol/1 -> Add/2
  InvalidValue/1 -> Add/1, DataTypeDuplicate/2, Add1/1
  Add1/1 -> Var_RelationalOper2/2
  Switch2/1 -> Y/1
  U/1 -> DataTypeDuplicate/1, Var_RelationalOper1/1, [in1]
  Logical_Operator12/1 -> Logical_Operator1/1
  tol1/1 -> Add1/2
  [in1] -> Var_RelationalOper2/1
  Var_RelationalOper1/1 -> Logical_Operator12/1
  [in1] -> Switch2/3
  Logical_Operator1/1 -> Switch2/2

== system Ampere_Library/User_Defined_Libraries/Signal_Routing/A_ExtDefaultValueSw ==
  note: Refer Mask Description of this Library block for detailed information.
  Inp1 : Inport
  Inp2 : Inport  Port=2
  Add : Sum  Inputs=+-  InputSameDT=on  OutDataTypeStr=Inherit: Inherit via back propagation  RndMeth=Zero
      settings: AttributesFormatString=SAT = %<SaturateOnIntegerOverflow>
  Add1 : Sum  InputSameDT=on  OutDataTypeStr=Inherit: Inherit via back propagation  RndMeth=Zero
      settings: AttributesFormatString=SAT = %<SaturateOnIntegerOverflow>
  DataTypeDuplicate : DataTypeDuplicate
  InvalidValue1 : Constant  Value=InvalidValue  OutDataTypeStr=Inherit: Inherit via back propagation
  Logical_Operator1 : Logic  Operator=NOT  OutDataTypeStr=boolean
  Logical_Operator4 : Logic  Operator=XOR  OutDataTypeStr=boolean
  Switch2 : Switch  Criteria=u2 ~= 0  RndMeth=Zero  SaturateOnIntegerOverflow=off
      settings: AttributesFormatString=SAT = %<SaturateOnIntegerOverflow>
  Var_RelationalOper1 : RelationalOperator  Operator=>  OutDataTypeStr=boolean  RndMeth=Zero
  Var_RelationalOper2 : RelationalOperator  Operator=<  OutDataTypeStr=boolean  RndMeth=Zero
  tol : Constant  Value=tol  OutDataTypeStr=Inherit: Inherit via back propagation
  tol1 : Constant  Value=tol  OutDataTypeStr=Inherit: Inherit via back propagation
  Y : Outport
  wires:
  [Inp2] -> Switch2/3
  Var_RelationalOper2/1 -> Logical_Operator4/2
  tol/1 -> Add/2
  Inp2/1 -> DataTypeDuplicate/1, Var_RelationalOper1/1, [Inp2]
  tol1/1 -> Add1/2
  InvalidValue1/1 -> DataTypeDuplicate/2, Add/1, Add1/1
  Inp1/1 -> Switch2/1
  Var_RelationalOper1/1 -> Logical_Operator4/1
  Add1/1 -> Var_RelationalOper2/2
  [Inp2] -> Var_RelationalOper2/1
  Logical_Operator4/1 -> Logical_Operator1/1
  Logical_Operator1/1 -> Switch2/2
  Switch2/1 -> Y/1
  Add/1 -> Var_RelationalOper1/2

== system Ampere_Library/User_Defined_Libraries/Signal_Routing/A_ResolutionBlock ==
  note: Rounding_system
  note: Refer Mask Description of this Library block for detailed information.
  U : Inport  OutDataTypeStr=double
      settings: AttributesFormatString=DT = %<OutDataTypeStr>
  Abs1 : Abs  RndMeth=Zero  SaturateOnIntegerOverflow=off
      settings: AttributesFormatString=SAT = %<SaturateOnIntegerOverflow>
  DataTypeConversion3 : DataTypeConversion  SaturateOnIntegerOverflow=off
  Product : Product  Inputs=*/  InputSameDT=on  RndMeth=Zero
  Product1 : Product  Inputs=**  InputSameDT=on  OutDataTypeStr=double  RndMeth=Zero
      settings: AttributesFormatString=|
      | DT = %<OutDataTypeStr>
      | SAT = %<SaturateOnIntegerOverflow>
  Product2 : Product  OutDataTypeStr=uint32  RndMeth=Zero  SaturateOnIntegerOverflow=on
      settings: AttributesFormatString=SAT = %<SaturateOnIntegerOverflow>\n DT = %<OutDataTypeStr>\n
  RF0 : Constant  Value=RF0
  RF05 : Constant  Value=RF05
  RF1 : Constant  Value=RF1
  RelationalOperator : RelationalOperator  Operator=>  OutDataTypeStr=boolean  RndMeth=Zero
  RelationalOperator1 : RelationalOperator  OutDataTypeStr=boolean  RndMeth=Zero
  RelationalOperator4 : RelationalOperator  OutDataTypeStr=boolean  RndMeth=Zero
  Resolution : Constant  Value=Resolution  OutDataTypeStr=Inherit: Inherit via back propagation
  Subtract1 : Sum  Inputs=-+  InputSameDT=on  RndMeth=Zero
  Subtract10 : Sum  Inputs=-+  InputSameDT=on  RndMeth=Zero
  Subtract2 : Sum  InputSameDT=on  RndMeth=Zero
  Subtract3 : Sum  Inputs=--  InputSameDT=on  RndMeth=Zero
  Switch{1..3,8..10} (6 alike) : Switch  Criteria=u2 ~= 0  RndMeth=Zero  SaturateOnIntegerOverflow=off
  Y : Outport
  wires:
  Switch10/1 -> Product1/1
  Product1/1 -> Y/1
  Resolution/1 -> Product1/2, Product/2
  U/1 -> Product/1
  [int_out] -> Subtract2/2
  RelationalOperator4/1 -> [Check]
  DataTypeConversion3/1 -> Subtract10/1, [int_out]
  Product2/1 -> DataTypeConversion3/1
  RF0/1 -> RelationalOperator4/2, [Zero_out]
  Product/1 -> Abs1/1, RelationalOperator4/1
  RF1/1 -> [cons1], Product2/1
  Abs1/1 -> Product2/2, Subtract10/2
  RelationalOperator1/1 -> Switch8/2, Switch9/2
  [Ceil_out] -> Switch8/1
  [Floor_out] -> Switch8/3
  [Floor_out] -> Switch9/1
  [Ceil_out] -> Switch9/3
  Switch8/1 -> Switch10/1
  Switch9/1 -> Switch10/3
  [Check] -> Switch10/2
  Subtract10/1 -> RelationalOperator1/1, RelationalOperator/1
  RF05/1 -> RelationalOperator1/2
  Subtract3/1 -> Switch1/3
  [Check] -> Switch1/2
  [Check] -> Switch2/2
  Subtract2/1 -> Switch2/1
  Switch2/1 -> [Ceil_out]
  Switch1/1 -> [Floor_out]
  Subtract1/1 -> Switch2/3
  [int_out] -> Subtract1/1
  [Zero_out] -> Subtract1/2
  [int_out] -> Switch1/1, Subtract3/1
  RelationalOperator/1 -> Switch3/2
  Switch3/1 -> Subtract3/2, Subtract2/1  "Diff_check"
  [Zero_out] -> Switch3/3, RelationalOperator/2
  [cons1] -> Switch3/1

== system Ampere_Library/User_Defined_Libraries/Signal_Routing/A_SlopeSwitch2Inputs ==
  note: Slope_On_Compute
  note: Detect Change
  note: Refer Mask Description of this Library block for detailed information.
  Switch_Cmd : Inport
  Pos_Slope : Inport  Port=2
  Neg_Slope : Inport  Port=3
  Inp0 : Inport  Port=4
  Inp1 : Inport  Port=5
  DataTypeConversion_19 : DataTypeConversion  OutDataTypeStr=uint8
      settings: AttributesFormatString=SAT = %<SaturateOnIntegerOverflow>
  LogicalOperator : Logic  Operator=OR  OutDataTypeStr=boolean
  Multiport_Switch : MultiPortSwitch  DataPortOrder=Zero-based contiguous  Inputs=2  DataPortForDefault=Additional data port  DiagnosticForDefault=None  zeroidx=on  RndMeth=Zero  SaturateOnIntegerOverflow=off
  Relational_Operator : RelationalOperator  Operator=~=  OutDataTypeStr=boolean  RndMeth=Zero
  Slope_On_Block : Subsystem
  Switch1 : Switch  Criteria=u2 ~= 0  RndMeth=Zero  SaturateOnIntegerOverflow=off
  Switch2 : Switch  Criteria=u2 ~= 0  RndMeth=Zero  SaturateOnIntegerOverflow=off
      settings: AttributesFormatString=SAT = %<SaturateOnIntegerOverflow>
  UnitDelay : UnitDelay  InitialCondition=InitDelay  SampleTime=-1  HasFrameUpgradeWarning=on
      settings: AttributesFormatString=Init = %<InitialCondition>\n
  UnitDelay1 : UnitDelay  InitialCondition=false  SampleTime=-1  HasFrameUpgradeWarning=on
      settings: AttributesFormatString=Init = %<InitialCondition>\n
  UnitDelay2 : UnitDelay  InitialCondition=InitDelay  SampleTime=-1  HasFrameUpgradeWarning=on
      settings: AttributesFormatString=Init = %<InitialCondition>\n
  UnitDelay3 : UnitDelay  InitialCondition=true  SampleTime=-1  HasFrameUpgradeWarning=on
      settings: AttributesFormatString=Init =%<InitialCondition>
  false : Constant  Value=false
  Out : Outport
  Slope_On : Outport  Port=2
  wires:
  Inp1/1 -> Multiport_Switch/3, Multiport_Switch/4
  false/1 -> UnitDelay3/1, Switch1/1
  Switch1/1 -> LogicalOperator/2
  UnitDelay/1 -> Relational_Operator/2
  UnitDelay3/1 -> Switch1/2
  [Inp] -> Switch2/3
  Pos_Slope/1 -> Slope_On_Block/2(Pos_Slope)
  [Slope_On] -> Switch2/2
  Inp0/1 -> Multiport_Switch/2
  UnitDelay2/1 -> Slope_On_Block/5(Prev_Output)  "Prev_Output"
  Slope_On_Block/2(Outp) -> Switch2/1
  Multiport_Switch/1 -> [Inp], Slope_On_Block/4(Inp)  "Inp"
  Neg_Slope/1 -> Slope_On_Block/3(Neg_Slope)
  DataTypeConversion_19/1 -> UnitDelay/1, Relational_Operator/1, Multiport_Switch/1
  UnitDelay1/1 -> LogicalOperator/1
  Switch2/1 -> Out/1, UnitDelay2/1
  Relational_Operator/1 -> Slope_On_Block/1(Signal_Change), Switch1/3  "Signal_Change"
  Slope_On_Block/1(Output_Not_Equals_Input) -> UnitDelay1/1
  LogicalOperator/1 -> Slope_On/1, [Slope_On], Slope_On_Block/Enable
  Switch_Cmd/1 -> DataTypeConversion_19/1

== system Ampere_Library/User_Defined_Libraries/Signal_Routing/A_TwoInDefltValSwitch ==
  note: Refer Mask Description of this Library block for detailed information.
  U1 : Inport
  U2 : Inport  Port=2
  Add : Sum  Inputs=+-  InputSameDT=on  RndMeth=Zero
      settings: AttributesFormatString=SAT = %<SaturateOnIntegerOverflow>
  Add1 : Sum  InputSameDT=on  RndMeth=Zero
      settings: AttributesFormatString=SAT = %<SaturateOnIntegerOverflow>
  DataTypeDuplicate : DataTypeDuplicate
  DefaultValue : Constant  Value=DefaultValue  OutDataTypeStr=Inherit: Inherit via back propagation
  InvalidValue : Constant  Value=InvalidValue  OutDataTypeStr=Inherit: Inherit via back propagation
  Logical_Operator1 : Logic  Operator=NOT  OutDataTypeStr=boolean
  Logical_Operator2 : Logic  Operator=XOR  OutDataTypeStr=boolean
  Switch2 : Switch  Criteria=u2 ~= 0  RndMeth=Zero  SaturateOnIntegerOverflow=off
      settings: AttributesFormatString=SAT = %<SaturateOnIntegerOverflow>
  Var_RelationalOper1 : RelationalOperator  Operator=>  OutDataTypeStr=boolean  RndMeth=Zero
  Var_RelationalOper2 : RelationalOperator  Operator=<  OutDataTypeStr=boolean  RndMeth=Zero
  tol : Constant  Value=tol  OutDataTypeStr=Inherit: Inherit via back propagation
  tol1 : Constant  Value=tol  OutDataTypeStr=Inherit: Inherit via back propagation
  Y : Outport
  wires:
  Add1/1 -> Var_RelationalOper2/2
  DefaultValue/1 -> Switch2/1
  Logical_Operator1/1 -> Switch2/2
  Add/1 -> Var_RelationalOper1/2
  Switch2/1 -> Y/1
  Logical_Operator2/1 -> Logical_Operator1/1
  tol/1 -> Add/2
  Var_RelationalOper1/1 -> Logical_Operator2/1
  [U2] -> Var_RelationalOper2/1
  U2/1 -> [U2], DataTypeDuplicate/1, Var_RelationalOper1/1
  tol1/1 -> Add1/2
  U1/1 -> Switch2/3
  InvalidValue/1 -> Add1/1, Add/1, DataTypeDuplicate/2
  Var_RelationalOper2/1 -> Logical_Operator2/2

== system Ampere_Library/User_Defined_Libraries/Signal_Routing/A_demux_fc ==
  note: This block is left for backwards compatibility. Function-call generator blocks are forbidden by LB001 rule. Users shall modify their models if this block is used.
  note: Refer Mask Description of this Library block for detailed information.
  fc_parent : TriggerPort  TriggerType=function-call  VariantControl=Variant
      settings: AttributesFormatString=%<StatesWhenEnabling>\n
  gen : S-Function  FunctionName=fcncallgen  Parameters=sample_time,numberOfIterations  SFunctionDeploymentMode=off  EnableBusSupport=off  mask(Function-Call Generator){sample_time=-1, numberOfIterations=1}
      mask prompts: sample_time "Simulink:masks:SampleTime_MP"; numberOfIterations "Simulink:masks:NumberOfIterations_MP"
      mask help: Simulink:masks:FunctionCallGenerator_MD
      mask init:
      | if ~isempty(numberOfIterations) & length(numberOfIterations) == 1 & (numberOfIterations > 1),
      | str=sprintf('iterate I = 1:%d',numberOfIterations);
      | else, str = 'f()';
      | end;
      mask Help: This block executes a function-call subsystem at the rate specified by the sample time and a specified number of times.
      mask DialogControl sample_time Prompt: Sample time:
      mask DialogControl numberOfIterations Prompt: Number of iterations:
      mask Display: disp(str)
  fc : Outport
  wires:
  gen/1 -> fc/1

== system Ampere_Library/User_Defined_Libraries/Sources/A_ClockGen ==
  note: Refer Mask Description of this Library block for detailed information.
  Sum1 : Sum  InputSameDT=on  RndMeth=Zero
      settings: AttributesFormatString=SAT = %<SaturateOnIntegerOverflow>
  UnitDelay : UnitDelay  InitialCondition=InitClock  SampleTime=-1  HasFrameUpgradeWarning=on
      settings: AttributesFormatString=Init = %<InitialCondition>
  st : Constant  Value=st  OutDataTypeStr=double
      settings: AttributesFormatString=DT = %<OutDataTypeStr>\n
  Out : Outport
  wires:
  UnitDelay/1 -> Out/1, Sum1/2
  st/1 -> Sum1/1
  Sum1/1 -> UnitDelay/1

== system Ampere_Library/User_Defined_Libraries/Sources/A_DownEdge_Event ==
  note: Refer Mask Description of this Library block for detailed information.
  Relational_Operator : RelationalOperator  Operator=<  OutDataTypeStr=boolean  RndMeth=Zero
  Unit_Delay : UnitDelay  InitialCondition=imm_clear  SampleTime=-1  HasFrameUpgradeWarning=on
      settings: AttributesFormatString=Init = %<InitialCondition>
  event_time : Constant  Value=event_time
  imm : Constant  Value=imm
  imm_clear : Constant  Value=imm_clear
  inclement : Sum  InputSameDT=on  RndMeth=Zero
  reset : Switch  Criteria=u2 ~= 0  RndMeth=Zero  SaturateOnIntegerOverflow=off
  sample_time : Constant  Value=sample_time
  target : Sum  InputSameDT=on  RndMeth=Zero
  target1 : Sum  Inputs=+-  InputSameDT=on  RndMeth=Zero
  event : Outport
  wires:
  target1/1 -> Relational_Operator/1
  sample_time/1 -> target1/2, inclement/1
  imm/1 -> target/2
  Relational_Operator/1 -> event/1, reset/2
  inclement/1 -> reset/3, Relational_Operator/2
  target/1 -> target1/1
  Unit_Delay/1 -> inclement/2
  event_time/1 -> target/1
  imm_clear/1 -> reset/1
  reset/1 -> Unit_Delay/1

== system Ampere_Library/User_Defined_Libraries/Sources/A_EnumConstant ==
  note: Refer Mask Description of this Library block for detailed information.
  Constant : Constant  Value=Ecst
  y : Outport
  wires:
  Constant/1 -> y/1
